simulink model "mayatnik"  (R2021b)
settings: Solver=VariableStepAuto  StartTime=0.0  StopTime=30  MaxStep=0.05  RelTol=1e-3
libraries: simulink_extras x1
settings Model: Creator=user  LastModifiedBy=user

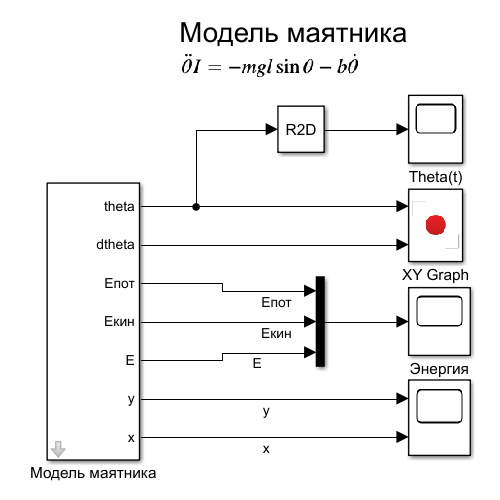
[thumbnail: Simulink's stored preview of the top-level diagram]
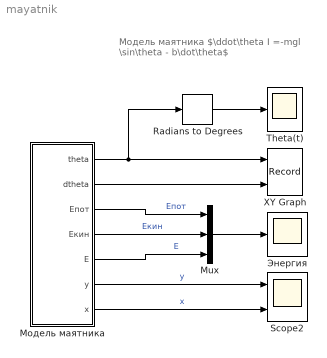
== system mayatnik ==
  note: Модель маятника
      | $\ddot\theta I =-mgl \sin\theta - b\dot\theta$
  Mux : Mux  Inputs=3
  Radians to Degrees : simulink_extras/Transformations/Radians to Degrees
  Scope2 : Scope  NumInputPorts=2
  Theta(t) : Scope
  XY Graph : Record  FileSettingsInternal="{\"entries\":[{\"content\":{\"excelSettings\":{\"content\":{},\"type\":\"Streamout.ExcelSettings\"}},\"type\":\"Streamout.FileSettingStorage\",\"uuid\":\"3e857f2d-5e14-4d25-91c5-5738f50bec84\"}],\"packageUris\":[\"http://schema.mathworks.com/mf0/streamout_blocks/R2020a\"],\"version\":\"1.0\"}"  Layout=[1 1]  SignalsInternal="{\"entries\":[{\"content\":{\"signals\":[{\"content\":{\"blockPath\":[\"mayatnik/XY Graph\"],\"channel\":[],\"dimensions\":[1],\"domain\":\"mayatnik/XY Graph\",\"lineColor\":\"#a2142f\",\"plots\":[1],\"port\":1,\"sid\":[\"\"],\"signalID\":556,\"signalName\":\"Модель маятника:1\"},\"type\":\"RecordBlkView.Signal\",\"uuid\":\"03f01e59-c0da-48ac-8aeb-1d450974e0f0\"},{\"content\":{\"blockPath\":[\"mayatnik/XY Graph\"],\"channel\":[],\"dimensions\":[1],\"domain\":\"mayatnik/XY Graph\",\"lineColor\":\"#139fff\",\"plots\":[1],\"port\":2,\"sid\":[\"\"],\"signalID\":560,\"signalName\":\"Модель маятника:2\"},\"type\":\"RecordBlkView.Signal\",\"uuid\":\"1c37eb2b-73fc-4784-8cc3-15cddaedb943\"}]},\"type\":\"RecordBlkView.InputSignals\",\"uuid\":\"b4adda22-86e8-4c50-9875-49ab3be24fdd\"}],\"packageUris\":[\"http://schema.mathworks.com/mf0/streamout_blocks/R2020a\"],\"version\":\"1.0\"}"  VisualizationBindings="{\"xyplotplugin\":{\"info\":[{\"series\":[{\"bindingParametersList\":[{\"parameter\":\"X-Axis\",\"signalID\":556,\"signalName\":\"РњРѕРґРµР»СЊ РјР°СЏС‚РЅРёРєР°:1\"},{\"parameter\":\"Y-Axis\",\"signalID\":560,\"signalName\":\"РњРѕРґРµР»СЊ РјР°СЏС‚РЅРёРєР°:2\"}],\"seriesID\":25440}],\"subplotID\":1}]}}"  CompatibilityTag=XY
  Модель маятника : Subsystem  mask{m=10, l=10, g=9.8, startDegree=30, b=0}
      mask prompts: m "масса"; l "длина подвеса"; g "ускорение свободного падения"; startDegree "стартовый угол"; b "диссипативный член"
      mask init:
      | I = m * l^2
  Энергия : Scope
  wires:
  Radians to Degrees/1 -> Theta(t)/1
  Модель маятника/1(theta) -> Radians to Degrees/1, XY Graph/1
  Модель маятника/2(dtheta) -> XY Graph/2
  Модель маятника/4(Екин) -> Mux/2  "Екин"
  Модель маятника/3(Eпот) -> Mux/1  "Eпот"
  Модель маятника/5(Е) -> Mux/3  "E"
  Mux/1 -> Энергия/1
  Модель маятника/6(y) -> Scope2/1  "y"
  Модель маятника/7(x) -> Scope2/2  "x"

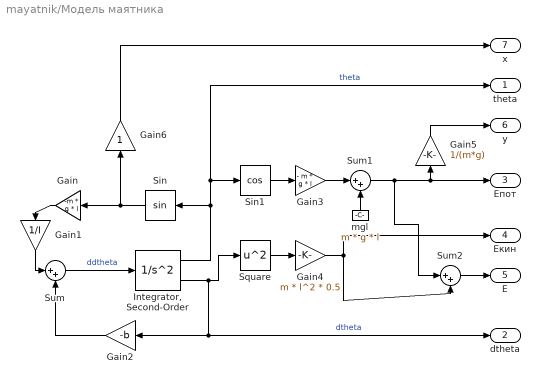
== system mayatnik/Модель маятника ==
  Gain : Gain  Gain=-m * g * l
  Gain1 : Gain  Gain=1/I
  Gain2 : Gain  Gain=-b
  Gain3 : Gain  Gain=- m * g * l
  Gain4 : Gain  Gain=m * l^2 * 0.5
  Gain5 : Gain  Gain=1/(m*g)
  Gain6 : Gain
  "Integrator, Second-Order" : SecondOrderIntegrator  ICX=deg2rad(startDegree)
  Sin : Trigonometry
  Sin1 : Trigonometry  Operator=cos
  Square : Math  Operator=square  SaturateOnIntegerOverflow=on
  Sum : Sum  Inputs=|++
  Sum1 : Sum  Inputs=|++
  Sum2 : Sum  Inputs=|++
  mgl : Constant  Value=m * g * l
  theta : Outport
  dtheta : Outport  Port=2
  Eпот : Outport  Port=3
  Екин : Outport  Port=4
  Е : Outport  Port=5
  y : Outport  Port=6
  x : Outport  Port=7
  wires:
  Sin/1 -> Gain/1, Gain6/1
  Gain/1 -> Gain1/1
  "Integrator, Second-Order"/1 -> Sin1/1, theta/1, Sin/1  "theta"
  "Integrator, Second-Order"/2 -> Gain2/1, dtheta/1, Square/1  "dtheta"
  Sum/1 -> "Integrator, Second-Order"/1  "ddtheta"
  Gain1/1 -> Sum/1
  Gain2/1 -> Sum/2
  Sin1/1 -> Gain3/1
  mgl/1 -> Sum1/2
  Gain3/1 -> Sum1/1
  Square/1 -> Gain4/1
  Gain4/1 -> Sum2/2, Екин/1
  Sum2/1 -> Е/1
  Sum1/1 -> Sum2/1, Gain5/1, Eпот/1
  Gain6/1 -> x/1
  Gain5/1 -> y/1
